simulink model "UPSControl"  (R2025b)
settings: Solver=VariableStepAuto  StartTime=0.0  StopTime=10  FixedStep=Ts  RelTol=1e-3
PostLoadFcn:
  | DataCenterParam;
values from neighbouring files (symbols this model uses):
  generator = struct    [GeneratorParam.m]
  lineInductance = 1e-6    (= 1e-06)    [DataCenterParam.m]    (also in GridParam.m)
  lineResistance = 1e-3    (= 0.001)    [DataCenterParam.m]    (also in GridParam.m)
  loadPower = 5e6    (= 5000000)    [DataCenterParam.m]    (also in LVRT.m; RedundancyAnalysis.m = 10000000)
  machine = struct    [GeneratorParam.m]
  powerTau = 0.005    [DataCenterParam.m]
  Ts = 5e-5    (= 5e-05)    [DataCenterParam.m]    (also in GeneratorParam.m)
  utilizationFactor = 0.45    [DataCenterParam.m]    (also in RedundancyAnalysis.m)
undefined symbols (not defined in the file or in its folder): breaker, ctLimitDelayTime, DiscIntNeverNeededParam, ee_sli_rtmsupport, gcbh, grid, rack, ups
libraries: nesl_utility x96, fl_lib x96, eeGeneralControl x84, ee_lib x80, simulink x68, eeTransforms x30, nesl_utility_internal x16, eeSinusoidalMeasurementV2 x13, slpidlib x12, simulink_extras x12, datacenter_lib x5, batteryecm_lib x4
(part 10 of 13)

== system UPSControl/Server Load/UPS Units/Single UPS/UPS/DC-Link/BESS/DC-DC Converter Controller/Current Reference Generator ==
  VoRef : Inport
  DischargeFlag : Inport  Port=2
  Vo : Inport  Port=3
  I : Inport  Port=4
  Mode : Inport  Port=5
  Add : Sum  Inputs=-+
  Gain : Gain  Gain=droopGain
  Low-Pass Filter (Discrete or Continuous) : eeGeneralControl/Low-Pass Filter (Discrete or Continuous)  K=1  T=0.001  B=inf  A=-inf  init_option=Inherited from block input  x0=0  Ts=-1
  PID Controller : slpidlib/PID Controller  Controller=PI  Form=Parallel  TimeDomain=Discrete-time  UseExternalTs=off  SampleTime=-1  IntegratorMethod=Forward Euler  FilterMethod=Forward Euler  ControllerParametersSource=internal  P=kpDC%500  I=kiDC%500  UseKiTs=off  D=0  UseExternalDerivativeSource=off  N=100  UseFilter=on  TunerSelectOption=Transfer Function Based (PID Tuner App)  InitialConditionSource=internal  InitialConditionForIntegrator=0  InitialConditionForFilter=0  DifferentiatorICPrevScaledInput=0  ExternalReset=rising  TrackingMode=off  Kt=1  LimitOutput=on  SatLimitsSource=internal  UpperSaturationLimit=0  LowerSaturationLimit=-5  LinearizeAsGain=on  AntiWindupMode=clamping  Kb=1  LimitIntegrator=off  UpperIntegratorSaturationLimit=4  LowerIntegratorSaturationLimit=-4  POutMin=[]  POutMax=[]  IOutMin=[]  IOutMax=[]  DOutMin=[]  DOutMax=[]  NOutMin=[]  NOutMax=[]  SumOutMin=[]  SumOutMax=[]  SaturationOutMin=[]  SaturationOutMax=[]  PParamMin=[]  PParamMax=[]  IParamMin=[]  IParamMax=[]  DParamMin=[]  DParamMax=[]  NParamMin=[]  NParamMax=[]  KbParamMin=[]  KbParamMax=[]  KtParamMin=[]  KtParamMax=[]  KbOutMin=[]  KbOutMax=[]  KtOutMin=[]  KtOutMax=[]  IntegratorOutMin=[]  IntegratorOutMax=[]  FilterOutMin=[]  FilterOutMax=[]  SumI1OutMin=[]  SumI1OutMax=[]  SumI2OutMin=[]  SumI2OutMax=[]  SumI3OutMin=[]  SumI3OutMax=[]  SumI4OutMin=[]  SumI4OutMax=[]  SumDOutMin=[]  SumDOutMax=[]  DifferentiatorOutMin=[]  DifferentiatorOutMax=[]  FilterDiffOutCoefMin=[]  FilterDiffOutCoefMax=[]  ReciprocalOutMin=[]  ReciprocalOutMax=[]  SumDenOutMin=[]  SumDenOutMax=[]  SumNumOutMin=[]  SumNumOutMax=[]  DivideOutMin=[]  DivideOutMax=[]  UdiffTsProdOutMin=[]  UdiffTsProdOutMax=[]  NTsProdOutMin=[]  NTsProdOutMax=[]  UintegralTsProdOutMin=[]  UintegralTsProdOutMax=[]  UngainTsProdOutMin=[]  UngainTsProdOutMax=[]  ClampingZeroOutDataTypeStr=Inherit: Inherit via back propagation  ClampingZeroOutMin=[]  ClampingZeroOutMax=[]  FilterDenConstantOutDataTypeStr=Inherit: Inherit via back propagation  FilterDenConstantOutMin=[]  FilterDenConstantOutMax=[]  PCopyOutDataTypeStr=Inherit: Inherit via back propagation  PCopyOutMin=[]  PCopyOutMax=[]  NCopyOutDataTypeStr=Inherit: Inherit via back propagation  NCopyOutMin=[]  NCopyOutMax=[]  IntegratorContinuousStateAttributes=''  IntegratorStateMustResolveToSignalObject=off  IntegratorRTWStateStorageClass=Auto  FilterContinuousStateAttributes=''  FilterStateMustResolveToSignalObject=off  FilterRTWStateStorageClass=Auto  ParallelPVariant=InternalParameters  IdealPVariant=Disabled  IVariant=InternalParameters  DVariant=Disabled  IntegratorVariant=Discrete  SatVariant=Enabled  AWVariant=DiscClampingParallel  PCopyVariant=Disabled  TRVariant=Disabled  FdbkBlocksVariant=Forward  IdealPFdbkVariant=Disabled  SatFdbkVariant=Disabled  DerivativeFilterVariant=Disabled  NVariant=Disabled  NCopyVariant=Disabled_SignalSpec  FilterICVariant=Disabled  IntegratorICVariant=InternalICs  ExternalResetVariant=ExternalReset  TRSumVariant=Passthrough  SumFdbkVariant=Disabled  SumVariant=Sum_PI  TsampFilterVariant=InternalTs  TsampNgainVariant=Passthrough  TsampIntegralVariant=Disabled_SignalSpec  ExternalSaturationOutDataTypeStr=Inherit: Same as second input  DerivativeSourceVariant=Disabled  PreIntVariant=InternalPreInt
  Saturation1 : Saturate  UpperLimit=0  LowerLimit=-10
  Switch1 : Switch  Criteria=u2 > Threshold  SaturateOnIntegerOverflow=off  InputSameDT=off
  Switch3 : Switch  Criteria=u2 > Threshold  SaturateOnIntegerOverflow=off  InputSameDT=off
  i : Outport  VectorParamsAs1DForOutWhenUnconnected=off
  wires:
  Switch1/1 -> Low-Pass Filter (Discrete or Continuous)/1
  Low-Pass Filter (Discrete or Continuous)/1 -> i/1
  Gain/1 -> Saturation1/1
  Switch3/1 -> Switch1/1
  Add/1 -> PID Controller/1, Gain/1
  VoRef/1 -> Add/1
  Vo/1 -> Add/2
  DischargeFlag/1 -> PID Controller/2, Switch1/2
  Mode/1 -> Switch3/2
  Saturation1/1 -> Switch3/1
  PID Controller/1 -> Switch3/3
  I/1 -> Switch1/3

== system UPSControl/Server Load/UPS Units/Single UPS/UPS/DC-Link/BESS/DC-DC Converter Controller/Mode Control ==
  iPFC : Inport
  Vdc : Inport  Port=2
  vBatt : Inport  Port=3
  vPCC : Inport  Port=4
  Breaker : Inport  Port=5
  iCharg : Inport  Port=6
  iBatt : Inport  Port=7
  BMS : Stateflow chart  TreatAsAtomicUnit=on  mask(Microgrid Transition and Dispatch Control){VMaxBatt=vBattMax, VdcRated=baseVoltageDC, iThreshold=vGridMin, iBattTh=10, vThreshold=0.9, VMaxDC=vDCThreshold, VBattNom=vBattMax, initialMode=initialMode}
      mask prompts: VMaxBatt "Maximum Battery Voltage (V)"; VdcRated "Rated DC bus voltage (V)"; iThreshold "Threshold mains current (A)"; iBattTh "Threshold battery current (A)"; vThreshold "Threshold mains voltage (V)"; VMaxDC "Threshold DC Bus Voltage (V)"; VBattNom "Battery nominal voltage (V)"; initialMode "Initial Operating Mode"
      mask help: This subsystem implements the transitions and the corresponding dispatch functions in the microgrid
  Compare To Constant : simulink/Logic and Bit Operations/Compare To Constant  relop===  const=4  OutDataTypeStr=boolean
  Constant : Constant  Value=0.98  OutDataTypeStr=double
  DischargeFlag : Outport
  vOut : Outport  Port=2
  iRef : Outport  Port=3
  droopMode : Outport  Port=4
  Mode : Outport  Port=5
  wires:
  iPFC/1 -> BMS/1(iPFC)
  Vdc/1 -> BMS/2(Vdc)
  vBatt/1 -> BMS/3(VBatt)
  Compare To Constant/1 -> DischargeFlag/1
  Constant/1 -> BMS/4(SOC)
  Breaker/1 -> BMS/5(breakerStatus)
  BMS/1(mode) -> Compare To Constant/1, Mode/1
  vPCC/1 -> BMS/6(VPCC)
  iCharg/1 -> BMS/7(iCharg)
  BMS/3(vOut) -> vOut/1
  BMS/2(iRef) -> iRef/1
  iBatt/1 -> BMS/8(iBatt)
  BMS/4(droopMode) -> droopMode/1

== system UPSControl/Server Load/UPS Units/Single UPS/UPS/Inverter/Filter & Measurements/PLL & Measurements/Measurement1 ==
  u : Inport
  Lead-Lag (Discrete or Continuous) : eeGeneralControl/Lead-Lag (Discrete or Continuous)  T1=0  T2=1e-3  B=inf  A=-inf  init_option=Inherited from block input  x0=0  Ts=Ts
  Vg : Outport
  wires:
  u/1 -> Lead-Lag (Discrete or Continuous)/1
  Lead-Lag (Discrete or Continuous)/1 -> Vg/1

== system UPSControl/Server Load/UPS Units/Single UPS/UPS/Inverter/Filter & Measurements/PLL & Measurements/Measurement2 ==
  u : Inport
  Lead-Lag (Discrete or Continuous) : eeGeneralControl/Lead-Lag (Discrete or Continuous)  T1=0  T2=1e-3  B=inf  A=-inf  init_option=Inherited from block input  x0=0  Ts=Ts
  Vg : Outport
  wires:
  u/1 -> Lead-Lag (Discrete or Continuous)/1
  Lead-Lag (Discrete or Continuous)/1 -> Vg/1

== system UPSControl/Server Load/UPS Units/Single UPS/UPS/Inverter/Filter & Measurements/PLL & Measurements/Subsystem ==
  Vabc : Inport
  Iabc : Inport  Port=2
  Add : Sum  Inputs=+-
  Constant : Constant  Value=pi/2
  Demux : Demux  Outputs=3
  Demux1 : Demux  Outputs=3
  Gain : Gain  Gain=1/frequency
  Gain1 : Gain  Gain=1/sqrt(2)
  Park Transform : eeTransforms/Park Transform  AxisAlignment=Q-axis  PowerInvariant=off
  Park Transform1 : eeTransforms/Park Transform  AxisAlignment=D-axis  PowerInvariant=off
  Scope : Scope  NumInputPorts=2
      settings: ActiveDisplayYMinimum=-0.205092135439717  ActiveDisplayYMaximum=1.5105061212865092  DataLoggingVariableName=ScopeData5
  Scope1 : Scope  NumInputPorts=2
      settings: ActiveDisplayYMinimum=-0.28974456970762869  ActiveDisplayYMaximum=0.89280252648921143  DataLoggingVariableName=ScopeData10
  Scope2 : Scope  NumInputPorts=2
      settings: ActiveDisplayYMinimum=-1  ActiveDisplayYMaximum=1  DataLoggingVariableName=ScopeData33
  Scope3 : Scope
      settings: ActiveDisplayYMinimum=-0.19602223868392757  ActiveDisplayYMaximum=1.7642001481553486  DataLoggingVariableName=ScopeData34
  "Sinusoidal Measurement (PLL, Three-Phase)" : eeSinusoidalMeasurementV2/Sinusoidal Measurement (PLL, Three-Phase)  InputFilter=on  InputNormalization=off  Kp_LF=40  Ki_LF=1000  F0=frequency  Theta0=0  Ts=Ts
  Terminator : Terminator
  Terminator1 : Terminator
  mag : Outport
  freq : Outport  Port=2
  angle : Outport  Port=3
  Vd : Outport  Port=4
  Vq : Outport  Port=5
  Id1 : Outport  Port=6
  Iq1 : Outport  Port=7
  wires:
  Iabc/1 -> Park Transform1/1
  Demux1/3 -> Terminator1/1
  Demux1/2 -> Scope1/2, Iq1/1
  Demux1/1 -> Scope1/1, Id1/1
  Park Transform1/1 -> Demux1/1
  "Sinusoidal Measurement (PLL, Three-Phase)"/3 -> Gain1/1
  "Sinusoidal Measurement (PLL, Three-Phase)"/1 -> Gain/1
  "Sinusoidal Measurement (PLL, Three-Phase)"/2 -> Park Transform/2, angle/1, Add/1
  Demux/2 -> Vq/1, Scope/2
  Demux/1 -> Vd/1, Scope/1
  Park Transform/1 -> Demux/1
  Vabc/1 -> Park Transform/1, "Sinusoidal Measurement (PLL, Three-Phase)"/1
  Demux/3 -> Terminator/1
  Gain/1 -> Scope2/1, freq/1
  Gain1/1 -> Scope3/1, mag/1
  Constant/1 -> Add/2
  Add/1 -> Park Transform1/2

== system UPSControl/Server Load/UPS Units/Single UPS/UPS/Inverter/Inverter Controller/Current Limiter/Current Limiter ==
  Igd : Inport
  Igq : Inport  Port=2
  Current Saturation : Subsystem  VariantControl=Current Saturation
  Virtual Impedance : Subsystem  VariantControl=Virtual Impedance
  delVd : Outport
  delVq : Outport  Port=2
  Idmax : Outport  Port=3
  Iqmax : Outport  Port=4

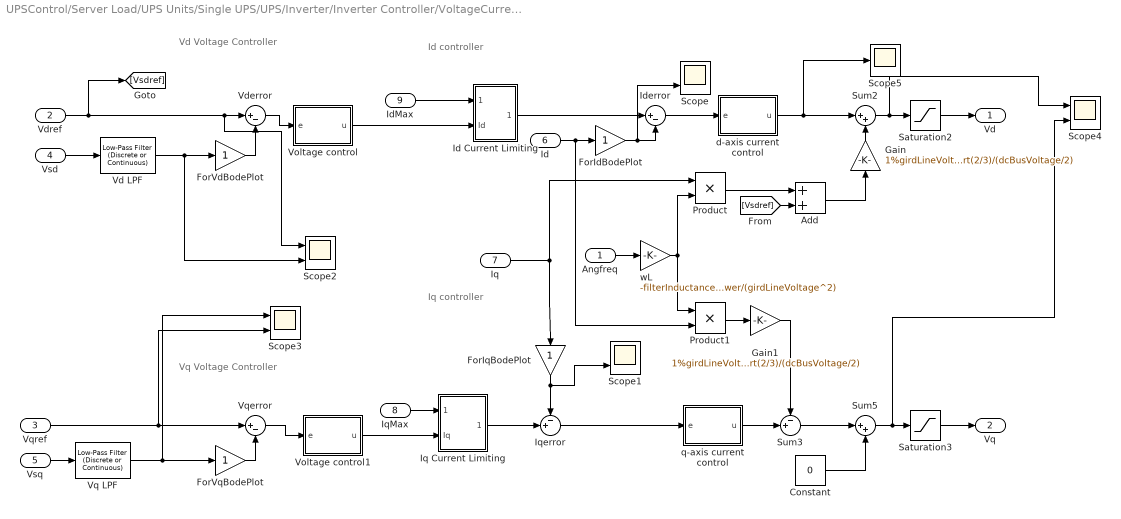
== system UPSControl/Server Load/UPS Units/Single UPS/UPS/Inverter/Inverter Controller/VoltageCurrentControl/Controller ==
  note: Vq Voltage Controller
  note: Iq controller
  note: Vd Voltage Controller
  note: Id controller
  Angfreq : Inport
  Vdref : Inport  Port=2
  Vqref : Inport  Port=3
  Vsd : Inport  Port=4
  Vsq : Inport  Port=5
  Id : Inport  Port=6
  Iq : Inport  Port=7
  IqMax : Inport  Port=8
  IdMax : Inport  Port=9
  Add : Sum
  Constant : Constant  Value=0  SampleTime=currentControlTs
  ForIdBodePlot : Gain
  ForIqBodePlot : Gain
  ForVdBodePlot : Gain
  ForVqBodePlot : Gain
  Gain : Gain  Gain=1%girdLineVoltage*sqrt(2/3)/(dcBusVoltage/2)
  Gain1 : Gain  Gain=1%girdLineVoltage*sqrt(2/3)/(dcBusVoltage/2)
  Id Current Limiting : Subsystem
  Iderror : Sum  Inputs=|+-
  Iq Current Limiting : Subsystem
  Iqerror : Sum  Inputs=-+|
  Product : Product
  Product1 : Product
  Saturation2 : Saturate  UpperLimit=1.5  LowerLimit=-1.5
  Saturation3 : Saturate  UpperLimit=1.5  LowerLimit=-1.5
  Scope{,1..4} (5 alike) : Scope  NumInputPorts=2
      Scope settings: ActiveDisplayYMinimum=-1.8047219913264509  ActiveDisplayYMaximum=2.2005246657029387
      Scope1 settings: ActiveDisplayYMinimum=-0.5206159009733754  ActiveDisplayYMaximum=0.33911481242712255
      Scope2 settings: ActiveDisplayYMinimum=0.98739217845302751  ActiveDisplayYMaximum=1.0346201805103583
      Scope3 settings: ActiveDisplayYMinimum=-1.1546814525903495  ActiveDisplayYMaximum=0.39213307331314629
      Scope4 settings: ActiveDisplayYMinimum=-0.18956095761758107  ActiveDisplayYMaximum=1.4204991580589943  DataLoggingVariableName=ScopeData41
  Scope5 : Scope
      settings: ActiveDisplayYMinimum=-1  ActiveDisplayYMaximum=1  DataLoggingVariableName=ScopeData42
  Sum2 : Sum  Inputs=|++
  Sum3 : Sum  Inputs=-+|
  Sum5 : Sum  Inputs=|++
  Vd LPF : eeGeneralControl/Low-Pass Filter (Discrete or Continuous)  K=1  T=vdvqLPFTimeConst  B=inf  A=-inf  init_option=Specify as parameter  x0=0  Ts=voltControlTs
  Vderror : Sum  Inputs=|+-
  Voltage control : Subsystem
  Voltage control1 : Subsystem
  Vq LPF : eeGeneralControl/Low-Pass Filter (Discrete or Continuous)  K=1  T=vdvqLPFTimeConst  B=inf  A=-inf  init_option=Inherited from block input  x0=0  Ts=voltControlTs
  Vqerror : Sum  Inputs=|+-
  d-axis current control : Subsystem
  q-axis current control : Subsystem
  wL : Gain  Gain=-filterInductance*power/(girdLineVoltage^2)
  Vd : Outport  VectorParamsAs1DForOutWhenUnconnected=off
  Vq : Outport  Port=2  VectorParamsAs1DForOutWhenUnconnected=off
  wires:
  Vdref/1 -> [Vsdref], Vderror/1, Scope2/1
  Vq LPF/1 -> ForVqBodePlot/1, Scope3/1
  Vd LPF/1 -> ForVdBodePlot/1, Scope2/2
  ForIqBodePlot/1 -> Iqerror/1, Scope1/2
  ForIdBodePlot/1 -> Iderror/2, Scope/2
  ForVqBodePlot/1 -> Vqerror/2
  ForVdBodePlot/1 -> Vderror/2
  Vsd/1 -> Vd LPF/1
  Gain/1 -> Sum2/2
  Add/1 -> Gain/1
  [Vsdref] -> Add/2
  Gain1/1 -> Sum3/1
  Vqerror/1 -> Voltage control1/1(e)
  Vqref/1 -> Vqerror/1, Scope3/2
  Vderror/1 -> Voltage control/1(e)
  Id/1 -> ForIdBodePlot/1, Product1/2
  Vsq/1 -> Vq LPF/1
  Sum5/1 -> Scope4/2, Saturation3/1
  Sum3/1 -> Sum5/1
  q-axis current control/1(u) -> Sum3/2
  Sum2/1 -> Scope4/1, Saturation2/1
  d-axis current control/1(u) -> Scope5/1, Sum2/1
  Product/1 -> Add/1
  Product1/1 -> Gain1/1
  Saturation2/1 -> Vd/1
  Saturation3/1 -> Vq/1
  Iderror/1 -> d-axis current control/1(e)
  Constant/1 -> Sum5/2
  Angfreq/1 -> wL/1
  wL/1 -> Product/2, Product1/1
  Iqerror/1 -> q-axis current control/1(e)
  Iq/1 -> Product/1, ForIqBodePlot/1
  IdMax/1 -> Id Current Limiting/1(Imax)
  IqMax/1 -> Iq Current Limiting/1(Imax)
  Voltage control/1(u) -> Id Current Limiting/2(Id)
  Id Current Limiting/1(Idref) -> Iderror/1
  Voltage control1/1(u) -> Iq Current Limiting/2(Iq)
  Iq Current Limiting/1(Iqref) -> Iqerror/2

== system UPSControl/Server Load/UPS Units/Single UPS/UPS/Inverter/Inverter Controller/VoltageCurrentControl/Modulation Signal ==
  Vd : Inport
  Vq : Inport  Port=2
  Angle : Inport  Port=3
  Constant : Constant  Value=0
  Constant1 : Constant  Value=1.05
  Inverse Park Transform : eeTransforms/Inverse Park Transform  AxisAlignment=D-axis  PowerInvariant=off
  Mux1 : Mux  Inputs=3
  Saturation : Saturate  UpperLimit=1.2  LowerLimit=-1.2
  Saturation1 : Saturate
  Saturation2 : Saturate  UpperLimit=1  LowerLimit=-1
  Scope : Scope  NumInputPorts=2
      settings: ActiveDisplayYMinimum=-1  ActiveDisplayYMaximum=1  DataLoggingVariableName=ScopeData9
  Scope1 : Scope
      settings: ActiveDisplayYMinimum=-1  ActiveDisplayYMaximum=1
  Scope2 : Scope
      settings: ActiveDisplayYMinimum=-1.25  ActiveDisplayYMaximum=1.25  DataLoggingVariableName=ScopeData47
  mabc : Outport  VectorParamsAs1DForOutWhenUnconnected=off
  wires:
  Vq/1 -> Saturation1/1, Scope/2
  Vd/1 -> Saturation/1, Scope/1
  Constant/1 -> Mux1/3
  Saturation2/1 -> Scope2/1, mabc/1
  Angle/1 -> Inverse Park Transform/2, Scope1/1
  Mux1/1 -> Inverse Park Transform/1
  Inverse Park Transform/1 -> Saturation2/1
  Saturation/1 -> Mux1/1
  Saturation1/1 -> Mux1/2

== system UPSControl/Server Load/UPS Units/Single UPS/UPS/Rectifier/PFC Rectifier Controller/Current Controller/Id and Iq Controller ==
  idRef : Inport
  iqRef : Inport  Port=2
  IdSens : Inport  Port=3
  iqSens : Inport  Port=4
  vd : Inport  Port=5
  vq : Inport  Port=6
  Reset : Inport  Port=7
  Constant4 : Constant  Value=0  SampleTime=Ts
  Gain1 : Gain  Gain=2*1*pi*Freq*L/BaseImpedance
  Gain2 : Gain  Gain=2*1*pi*Freq*L/BaseImpedance
  IdPID : slpidlib/PID Controller  Controller=PID  Form=Parallel  TimeDomain=Discrete-time  UseExternalTs=off  SampleTime=Ts  IntegratorMethod=Forward Euler  FilterMethod=Forward Euler  ControllerParametersSource=internal  P=KpdCurrent  I=KidCurrent  UseKiTs=off  D=KddCurrent  UseExternalDerivativeSource=off  N=NdCurrent  UseFilter=on  TunerSelectOption=Transfer Function Based (PID Tuner App)  InitialConditionSource=internal  InitialConditionForIntegrator=0  InitialConditionForFilter=0  DifferentiatorICPrevScaledInput=0  ExternalReset=falling  TrackingMode=off  Kt=1  LimitOutput=on  SatLimitsSource=internal  UpperSaturationLimit=IdControlUpperLimit  LowerSaturationLimit=IdControlLowerLimit  LinearizeAsGain=on  AntiWindupMode=clamping  Kb=1  LimitIntegrator=on  UpperIntegratorSaturationLimit=IdControlUpperLimit  LowerIntegratorSaturationLimit=IdControlLowerLimit  POutMin=[]  POutMax=[]  IOutMin=[]  IOutMax=[]  DOutMin=[]  DOutMax=[]  NOutMin=[]  NOutMax=[]  SumOutMin=[]  SumOutMax=[]  SaturationOutMin=[]  SaturationOutMax=[]  PParamMin=[]  PParamMax=[]  IParamMin=[]  IParamMax=[]  DParamMin=[]  DParamMax=[]  NParamMin=[]  NParamMax=[]  KbParamMin=[]  KbParamMax=[]  KtParamMin=[]  KtParamMax=[]  KbOutMin=[]  KbOutMax=[]  KtOutMin=[]  KtOutMax=[]  IntegratorOutMin=[]  IntegratorOutMax=[]  FilterOutMin=[]  FilterOutMax=[]  SumI1OutMin=[]  SumI1OutMax=[]  SumI2OutMin=[]  SumI2OutMax=[]  SumI3OutMin=[]  SumI3OutMax=[]  SumI4OutMin=[]  SumI4OutMax=[]  SumDOutMin=[]  SumDOutMax=[]  DifferentiatorOutMin=[]  DifferentiatorOutMax=[]  FilterDiffOutCoefMin=[]  FilterDiffOutCoefMax=[]  ReciprocalOutMin=[]  ReciprocalOutMax=[]  SumDenOutMin=[]  SumDenOutMax=[]  SumNumOutMin=[]  SumNumOutMax=[]  DivideOutMin=[]  DivideOutMax=[]  UdiffTsProdOutMin=[]  UdiffTsProdOutMax=[]  NTsProdOutMin=[]  NTsProdOutMax=[]  UintegralTsProdOutMin=[]  UintegralTsProdOutMax=[]  UngainTsProdOutMin=[]  UngainTsProdOutMax=[]  ClampingZeroOutDataTypeStr=Inherit: Inherit via back propagation  ClampingZeroOutMin=[]  ClampingZeroOutMax=[]  FilterDenConstantOutDataTypeStr=Inherit: Inherit via back propagation  FilterDenConstantOutMin=[]  FilterDenConstantOutMax=[]  PCopyOutDataTypeStr=Inherit: Inherit via back propagation  PCopyOutMin=[]  PCopyOutMax=[]  NCopyOutDataTypeStr=Inherit: Inherit via back propagation  NCopyOutMin=[]  NCopyOutMax=[]  IntegratorContinuousStateAttributes=''  IntegratorStateMustResolveToSignalObject=off  IntegratorRTWStateStorageClass=Auto  FilterContinuousStateAttributes=''  FilterStateMustResolveToSignalObject=off  FilterRTWStateStorageClass=Auto  ParallelPVariant=InternalParameters  IdealPVariant=Disabled  IVariant=InternalParameters  DVariant=InternalParameters  IntegratorVariant=Discrete  SatVariant=Enabled  AWVariant=DiscClampingParallel  PCopyVariant=Disabled  TRVariant=Disabled  FdbkBlocksVariant=Forward  IdealPFdbkVariant=Disabled  SatFdbkVariant=Disabled  DerivativeFilterVariant=ForwardEulerFilter  NVariant=InternalParameters  NCopyVariant=Disabled  FilterICVariant=InternalICsFilter  IntegratorICVariant=InternalICs  ExternalResetVariant=ExternalReset  TRSumVariant=Passthrough  SumFdbkVariant=Disabled  SumVariant=Sum_PID  TsampFilterVariant=InternalTs  TsampNgainVariant=Passthrough  TsampIntegralVariant=Disabled_SignalSpec  ExternalSaturationOutDataTypeStr=Inherit: Same as second input  DerivativeSourceVariant=ErrorSignal  PreIntVariant=InternalPreInt
  IqPID : slpidlib/PID Controller  Controller=PID  Form=Parallel  TimeDomain=Discrete-time  UseExternalTs=off  SampleTime=Ts  IntegratorMethod=Forward Euler  FilterMethod=Forward Euler  ControllerParametersSource=internal  P=KpqCurrent  I=KiqCurrent  UseKiTs=off  D=KdqCurrent  UseExternalDerivativeSource=off  N=NdCurrent  UseFilter=on  TunerSelectOption=Transfer Function Based (PID Tuner App)  InitialConditionSource=internal  InitialConditionForIntegrator=0  InitialConditionForFilter=0  DifferentiatorICPrevScaledInput=0  ExternalReset=falling  TrackingMode=off  Kt=1  LimitOutput=on  SatLimitsSource=internal  UpperSaturationLimit=IqControlUpperLimit  LowerSaturationLimit=IqControlLowerLimit  LinearizeAsGain=on  AntiWindupMode=clamping  Kb=1  LimitIntegrator=on  UpperIntegratorSaturationLimit=IqControlUpperLimit  LowerIntegratorSaturationLimit=IqControlLowerLimit  POutMin=[]  POutMax=[]  IOutMin=[]  IOutMax=[]  DOutMin=[]  DOutMax=[]  NOutMin=[]  NOutMax=[]  SumOutMin=[]  SumOutMax=[]  SaturationOutMin=[]  SaturationOutMax=[]  PParamMin=[]  PParamMax=[]  IParamMin=[]  IParamMax=[]  DParamMin=[]  DParamMax=[]  NParamMin=[]  NParamMax=[]  KbParamMin=[]  KbParamMax=[]  KtParamMin=[]  KtParamMax=[]  KbOutMin=[]  KbOutMax=[]  KtOutMin=[]  KtOutMax=[]  IntegratorOutMin=[]  IntegratorOutMax=[]  FilterOutMin=[]  FilterOutMax=[]  SumI1OutMin=[]  SumI1OutMax=[]  SumI2OutMin=[]  SumI2OutMax=[]  SumI3OutMin=[]  SumI3OutMax=[]  SumI4OutMin=[]  SumI4OutMax=[]  SumDOutMin=[]  SumDOutMax=[]  DifferentiatorOutMin=[]  DifferentiatorOutMax=[]  FilterDiffOutCoefMin=[]  FilterDiffOutCoefMax=[]  ReciprocalOutMin=[]  ReciprocalOutMax=[]  SumDenOutMin=[]  SumDenOutMax=[]  SumNumOutMin=[]  SumNumOutMax=[]  DivideOutMin=[]  DivideOutMax=[]  UdiffTsProdOutMin=[]  UdiffTsProdOutMax=[]  NTsProdOutMin=[]  NTsProdOutMax=[]  UintegralTsProdOutMin=[]  UintegralTsProdOutMax=[]  UngainTsProdOutMin=[]  UngainTsProdOutMax=[]  ClampingZeroOutDataTypeStr=Inherit: Inherit via back propagation  ClampingZeroOutMin=[]  ClampingZeroOutMax=[]  FilterDenConstantOutDataTypeStr=Inherit: Inherit via back propagation  FilterDenConstantOutMin=[]  FilterDenConstantOutMax=[]  PCopyOutDataTypeStr=Inherit: Inherit via back propagation  PCopyOutMin=[]  PCopyOutMax=[]  NCopyOutDataTypeStr=Inherit: Inherit via back propagation  NCopyOutMin=[]  NCopyOutMax=[]  IntegratorContinuousStateAttributes=''  IntegratorStateMustResolveToSignalObject=off  IntegratorRTWStateStorageClass=Auto  FilterContinuousStateAttributes=''  FilterStateMustResolveToSignalObject=off  FilterRTWStateStorageClass=Auto  ParallelPVariant=InternalParameters  IdealPVariant=Disabled  IVariant=InternalParameters  DVariant=InternalParameters  IntegratorVariant=Discrete  SatVariant=Enabled  AWVariant=DiscClampingParallel  PCopyVariant=Disabled  TRVariant=Disabled  FdbkBlocksVariant=Forward  IdealPFdbkVariant=Disabled  SatFdbkVariant=Disabled  DerivativeFilterVariant=ForwardEulerFilter  NVariant=InternalParameters  NCopyVariant=Disabled  FilterICVariant=InternalICsFilter  IntegratorICVariant=InternalICs  ExternalResetVariant=ExternalReset  TRSumVariant=Passthrough  SumFdbkVariant=Disabled  SumVariant=Sum_PID  TsampFilterVariant=InternalTs  TsampNgainVariant=Passthrough  TsampIntegralVariant=Disabled_SignalSpec  ExternalSaturationOutDataTypeStr=Inherit: Same as second input  DerivativeSourceVariant=ErrorSignal  PreIntVariant=InternalPreInt
  Mux1 : Mux  Inputs=3
  Sum1 : Sum  Inputs=|+-
  Sum2 : Sum  Inputs=|+-+
  Sum4 : Sum  Inputs=|--+
  Sum5 : Sum  Inputs=|+-
  vdqoRef : Outport
  IdCntrlError : Outport  Port=2
  IqCntrlError : Outport  Port=3
  wires:
  iqRef/1 -> Sum5/1
  Mux1/1 -> vdqoRef/1
  idRef/1 -> Sum1/1
  IqPID/1 -> Sum4/2
  IdSens/1 -> Gain1/1, Sum1/2
  Sum1/1 -> IdPID/1, IdCntrlError/1
  vd/1 -> Sum2/1
  IdPID/1 -> Sum2/2
  Gain2/1 -> Sum2/3
  Gain1/1 -> Sum4/1
  vq/1 -> Sum4/3
  iqSens/1 -> Gain2/1, Sum5/2
  Sum2/1 -> Mux1/1
  Sum4/1 -> Mux1/2
  Sum5/1 -> IqPID/1, IqCntrlError/1
  Constant4/1 -> Mux1/3
  Reset/1 -> IqPID/2, IdPID/2

== system UPSControl/Server Load/UPS Units/Single UPS/UPS/Rectifier/PFC Rectifier Controller/DC Voltage Controller and Current Reference/Iq Reference ==
  V_mag : Inport
  Q_ref : Inport  Port=2
  Divide2 : Product  Inputs=*/
  iq_ref : Outport
  wires:
  V_mag/1 -> Divide2/2
  Q_ref/1 -> Divide2/1
  Divide2/1 -> iq_ref/1

== system UPSControl/Server Load/UPS Units/Single UPS/UPS/Rectifier/PFC Rectifier Controller/DC Voltage Controller and Current Reference/Voltage Controller ==
  Vdcref : Inport
  Vdcmeas : Inport  Port=2
  Reset : Inport  Port=3
  Gain : Gain  Gain=1/BaseVdc
  Saturation : Saturate  UpperLimit=IdRefUpperLimit  LowerLimit=0
  Sum : Sum  Inputs=|+-
  Voltage control : Subsystem
  Id : Outport
  wires:
  Sum/1 -> Gain/1
  Gain/1 -> Voltage control/1(e)
  Vdcmeas/1 -> Sum/2
  Vdcref/1 -> Sum/1
  Voltage control/1(u) -> Saturation/1
  Saturation/1 -> Id/1
  Reset/1 -> Voltage control/2(Reset)

== system UPSControl/Server Load/UPS Units/Three UPS Parallel/UPS1/DC-Link/BESS/DC-DC Converter Controller/Current Reference Generator ==
  VoRef : Inport
  DischargeFlag : Inport  Port=2
  Vo : Inport  Port=3
  I : Inport  Port=4
  Mode : Inport  Port=5
  Add : Sum  Inputs=-+
  Gain : Gain  Gain=droopGain
  Low-Pass Filter (Discrete or Continuous) : eeGeneralControl/Low-Pass Filter (Discrete or Continuous)  K=1  T=0.001  B=inf  A=-inf  init_option=Inherited from block input  x0=0  Ts=-1
  PID Controller : slpidlib/PID Controller  Controller=PI  Form=Parallel  TimeDomain=Discrete-time  UseExternalTs=off  SampleTime=-1  IntegratorMethod=Forward Euler  FilterMethod=Forward Euler  ControllerParametersSource=internal  P=kpDC  I=kiDC*10  UseKiTs=off  D=0  UseExternalDerivativeSource=off  N=100  UseFilter=on  TunerSelectOption=Transfer Function Based (PID Tuner App)  InitialConditionSource=internal  InitialConditionForIntegrator=0  InitialConditionForFilter=0  DifferentiatorICPrevScaledInput=0  ExternalReset=rising  TrackingMode=off  Kt=1  LimitOutput=on  SatLimitsSource=internal  UpperSaturationLimit=0  LowerSaturationLimit=-5  LinearizeAsGain=on  AntiWindupMode=clamping  Kb=1  LimitIntegrator=off  UpperIntegratorSaturationLimit=4  LowerIntegratorSaturationLimit=-4  POutMin=[]  POutMax=[]  IOutMin=[]  IOutMax=[]  DOutMin=[]  DOutMax=[]  NOutMin=[]  NOutMax=[]  SumOutMin=[]  SumOutMax=[]  SaturationOutMin=[]  SaturationOutMax=[]  PParamMin=[]  PParamMax=[]  IParamMin=[]  IParamMax=[]  DParamMin=[]  DParamMax=[]  NParamMin=[]  NParamMax=[]  KbParamMin=[]  KbParamMax=[]  KtParamMin=[]  KtParamMax=[]  KbOutMin=[]  KbOutMax=[]  KtOutMin=[]  KtOutMax=[]  IntegratorOutMin=[]  IntegratorOutMax=[]  FilterOutMin=[]  FilterOutMax=[]  SumI1OutMin=[]  SumI1OutMax=[]  SumI2OutMin=[]  SumI2OutMax=[]  SumI3OutMin=[]  SumI3OutMax=[]  SumI4OutMin=[]  SumI4OutMax=[]  SumDOutMin=[]  SumDOutMax=[]  DifferentiatorOutMin=[]  DifferentiatorOutMax=[]  FilterDiffOutCoefMin=[]  FilterDiffOutCoefMax=[]  ReciprocalOutMin=[]  ReciprocalOutMax=[]  SumDenOutMin=[]  SumDenOutMax=[]  SumNumOutMin=[]  SumNumOutMax=[]  DivideOutMin=[]  DivideOutMax=[]  UdiffTsProdOutMin=[]  UdiffTsProdOutMax=[]  NTsProdOutMin=[]  NTsProdOutMax=[]  UintegralTsProdOutMin=[]  UintegralTsProdOutMax=[]  UngainTsProdOutMin=[]  UngainTsProdOutMax=[]  ClampingZeroOutDataTypeStr=Inherit: Inherit via back propagation  ClampingZeroOutMin=[]  ClampingZeroOutMax=[]  FilterDenConstantOutDataTypeStr=Inherit: Inherit via back propagation  FilterDenConstantOutMin=[]  FilterDenConstantOutMax=[]  PCopyOutDataTypeStr=Inherit: Inherit via back propagation  PCopyOutMin=[]  PCopyOutMax=[]  NCopyOutDataTypeStr=Inherit: Inherit via back propagation  NCopyOutMin=[]  NCopyOutMax=[]  IntegratorContinuousStateAttributes=''  IntegratorStateMustResolveToSignalObject=off  IntegratorRTWStateStorageClass=Auto  FilterContinuousStateAttributes=''  FilterStateMustResolveToSignalObject=off  FilterRTWStateStorageClass=Auto  ParallelPVariant=InternalParameters  IdealPVariant=Disabled  IVariant=InternalParameters  DVariant=Disabled  IntegratorVariant=Discrete  SatVariant=Enabled  AWVariant=DiscClampingParallel  PCopyVariant=Disabled  TRVariant=Disabled  FdbkBlocksVariant=Forward  IdealPFdbkVariant=Disabled  SatFdbkVariant=Disabled  DerivativeFilterVariant=Disabled  NVariant=Disabled  NCopyVariant=Disabled_SignalSpec  FilterICVariant=Disabled  IntegratorICVariant=InternalICs  ExternalResetVariant=ExternalReset  TRSumVariant=Passthrough  SumFdbkVariant=Disabled  SumVariant=Sum_PI  TsampFilterVariant=InternalTs  TsampNgainVariant=Passthrough  TsampIntegralVariant=Disabled_SignalSpec  ExternalSaturationOutDataTypeStr=Inherit: Same as second input  DerivativeSourceVariant=Disabled  PreIntVariant=InternalPreInt
  Saturation1 : Saturate  UpperLimit=0  LowerLimit=-10
  Switch1 : Switch  Criteria=u2 > Threshold  SaturateOnIntegerOverflow=off  InputSameDT=off
  Switch3 : Switch  Criteria=u2 > Threshold  SaturateOnIntegerOverflow=off  InputSameDT=off
  i : Outport  VectorParamsAs1DForOutWhenUnconnected=off
  wires:
  Switch1/1 -> Low-Pass Filter (Discrete or Continuous)/1
  Low-Pass Filter (Discrete or Continuous)/1 -> i/1
  Gain/1 -> Saturation1/1
  Switch3/1 -> Switch1/1
  Add/1 -> PID Controller/1, Gain/1
  VoRef/1 -> Add/1
  Vo/1 -> Add/2
  DischargeFlag/1 -> PID Controller/2, Switch1/2
  Mode/1 -> Switch3/2
  Saturation1/1 -> Switch3/1
  PID Controller/1 -> Switch3/3
  I/1 -> Switch1/3

== system UPSControl/Server Load/UPS Units/Three UPS Parallel/UPS1/DC-Link/BESS/DC-DC Converter Controller/Mode Control ==
  iPFC : Inport
  Vdc : Inport  Port=2
  vBatt : Inport  Port=3
  vPCC : Inport  Port=4
  Breaker : Inport  Port=5
  iCharg : Inport  Port=6
  iBatt : Inport  Port=7
  BMS : Stateflow chart  TreatAsAtomicUnit=on  mask(Microgrid Transition and Dispatch Control){VMaxBatt=vBattMax, VdcRated=baseVoltageDC, iThreshold=vGridMin, iBattTh=10, vThreshold=0.9, VMaxDC=vDCThreshold, VBattNom=vBattMax, initialMode=initialMode}
      mask prompts: VMaxBatt "Maximum Battery Voltage (V)"; VdcRated "Rated DC bus voltage (V)"; iThreshold "Threshold mains current (A)"; iBattTh "Threshold battery current (A)"; vThreshold "Threshold mains voltage (V)"; VMaxDC "Threshold DC Bus Voltage (V)"; VBattNom "Battery nominal voltage (V)"; initialMode "Initial Operating Mode"
      mask help: This subsystem implements the transitions and the corresponding dispatch functions in the microgrid
  Compare To Constant : simulink/Logic and Bit Operations/Compare To Constant  relop===  const=4  OutDataTypeStr=boolean
  Constant : Constant  Value=0.98  OutDataTypeStr=double
  DischargeFlag : Outport
  vOut : Outport  Port=2
  iRef : Outport  Port=3
  droopMode : Outport  Port=4
  Mode : Outport  Port=5
  wires:
  iPFC/1 -> BMS/1(iPFC)
  Vdc/1 -> BMS/2(Vdc)
  vBatt/1 -> BMS/3(VBatt)
  Compare To Constant/1 -> DischargeFlag/1
  Constant/1 -> BMS/4(SOC)
  Breaker/1 -> BMS/5(breakerStatus)
  BMS/1(mode) -> Compare To Constant/1, Mode/1
  vPCC/1 -> BMS/6(VPCC)
  iCharg/1 -> BMS/7(iCharg)
  BMS/3(vOut) -> vOut/1
  BMS/2(iRef) -> iRef/1
  iBatt/1 -> BMS/8(iBatt)
  BMS/4(droopMode) -> droopMode/1

== system UPSControl/Server Load/UPS Units/Three UPS Parallel/UPS1/Inverter/Filter & Measurements/PLL & Measurements/Measurement1 ==
  u : Inport
  Lead-Lag (Discrete or Continuous) : eeGeneralControl/Lead-Lag (Discrete or Continuous)  T1=0  T2=1e-3  B=inf  A=-inf  init_option=Inherited from block input  x0=0  Ts=Ts
  Vg : Outport
  wires:
  u/1 -> Lead-Lag (Discrete or Continuous)/1
  Lead-Lag (Discrete or Continuous)/1 -> Vg/1

== system UPSControl/Server Load/UPS Units/Three UPS Parallel/UPS1/Inverter/Filter & Measurements/PLL & Measurements/Measurement2 ==
  u : Inport
  Lead-Lag (Discrete or Continuous) : eeGeneralControl/Lead-Lag (Discrete or Continuous)  T1=0  T2=1e-3  B=inf  A=-inf  init_option=Inherited from block input  x0=0  Ts=Ts
  Vg : Outport
  wires:
  u/1 -> Lead-Lag (Discrete or Continuous)/1
  Lead-Lag (Discrete or Continuous)/1 -> Vg/1

== system UPSControl/Server Load/UPS Units/Three UPS Parallel/UPS1/Inverter/Filter & Measurements/PLL & Measurements/Subsystem ==
  Vabc : Inport
  Iabc : Inport  Port=2
  Add : Sum  Inputs=+-
  Constant : Constant  Value=pi/2
  Demux : Demux  Outputs=3
  Demux1 : Demux  Outputs=3
  Gain : Gain  Gain=1/frequency
  Gain1 : Gain  Gain=1/sqrt(2)
  Park Transform : eeTransforms/Park Transform  AxisAlignment=Q-axis  PowerInvariant=off
  Park Transform1 : eeTransforms/Park Transform  AxisAlignment=D-axis  PowerInvariant=off
  Scope : Scope  NumInputPorts=2
      settings: ActiveDisplayYMinimum=-0.205092135439717  ActiveDisplayYMaximum=1.5105061212865092  DataLoggingVariableName=ScopeData5
  Scope1 : Scope  NumInputPorts=2
      settings: ActiveDisplayYMinimum=-0.28974456970762869  ActiveDisplayYMaximum=0.89280252648921143  DataLoggingVariableName=ScopeData10
  Scope2 : Scope  NumInputPorts=2
      settings: ActiveDisplayYMinimum=-1  ActiveDisplayYMaximum=1  DataLoggingVariableName=ScopeData33
  Scope3 : Scope
      settings: ActiveDisplayYMinimum=-0.19602223868392757  ActiveDisplayYMaximum=1.7642001481553486  DataLoggingVariableName=ScopeData34
  "Sinusoidal Measurement (PLL, Three-Phase)" : eeSinusoidalMeasurementV2/Sinusoidal Measurement (PLL, Three-Phase)  InputFilter=on  InputNormalization=off  Kp_LF=40  Ki_LF=1000  F0=frequency  Theta0=0  Ts=Ts
  Terminator : Terminator
  Terminator1 : Terminator
  mag : Outport
  freq : Outport  Port=2
  angle : Outport  Port=3
  Vd : Outport  Port=4
  Vq : Outport  Port=5
  Id1 : Outport  Port=6
  Iq1 : Outport  Port=7
  wires:
  Iabc/1 -> Park Transform1/1
  Demux1/3 -> Terminator1/1
  Demux1/2 -> Scope1/2, Iq1/1
  Demux1/1 -> Scope1/1, Id1/1
  Park Transform1/1 -> Demux1/1
  "Sinusoidal Measurement (PLL, Three-Phase)"/3 -> Gain1/1
  "Sinusoidal Measurement (PLL, Three-Phase)"/1 -> Gain/1
  "Sinusoidal Measurement (PLL, Three-Phase)"/2 -> Park Transform/2, angle/1, Add/1
  Demux/2 -> Vq/1, Scope/2
  Demux/1 -> Vd/1, Scope/1
  Park Transform/1 -> Demux/1
  Vabc/1 -> Park Transform/1, "Sinusoidal Measurement (PLL, Three-Phase)"/1
  Demux/3 -> Terminator/1
  Gain/1 -> Scope2/1, freq/1
  Gain1/1 -> Scope3/1, mag/1
  Constant/1 -> Add/2
  Add/1 -> Park Transform1/2

== system UPSControl/Server Load/UPS Units/Three UPS Parallel/UPS1/Inverter/Inverter Controller/Current Limiter/Current Limiter ==
  Igd : Inport
  Igq : Inport  Port=2
  Current Saturation : Subsystem  VariantControl=Current Saturation
  Virtual Impedance : Subsystem  VariantControl=Virtual Impedance
  delVd : Outport
  delVq : Outport  Port=2
  Idmax : Outport  Port=3
  Iqmax : Outport  Port=4

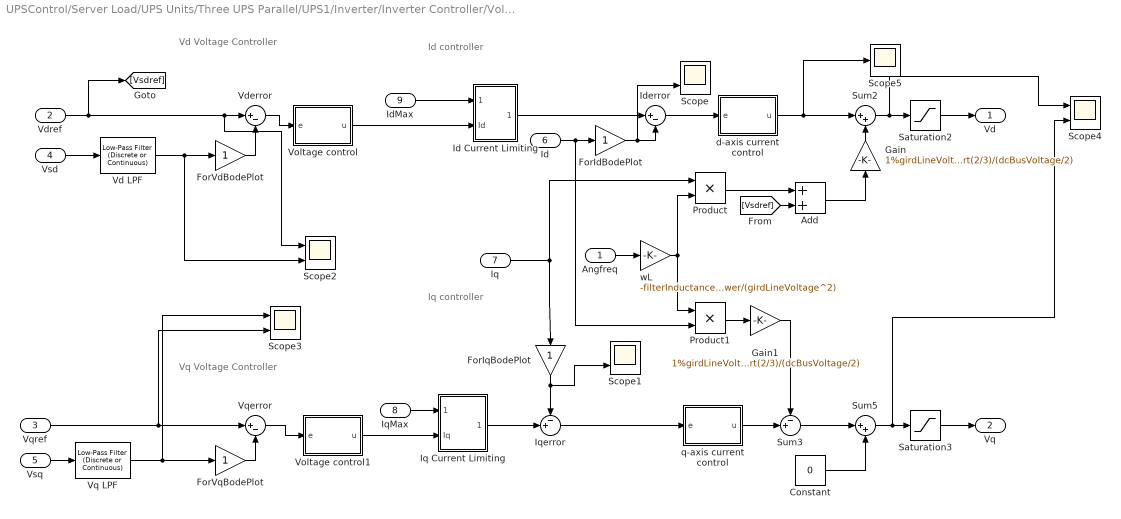
== system UPSControl/Server Load/UPS Units/Three UPS Parallel/UPS1/Inverter/Inverter Controller/VoltageCurrentControl/Controller ==
  note: Vq Voltage Controller
  note: Iq controller
  note: Vd Voltage Controller
  note: Id controller
  Angfreq : Inport
  Vdref : Inport  Port=2
  Vqref : Inport  Port=3
  Vsd : Inport  Port=4
  Vsq : Inport  Port=5
  Id : Inport  Port=6
  Iq : Inport  Port=7
  IqMax : Inport  Port=8
  IdMax : Inport  Port=9
  Add : Sum
  Constant : Constant  Value=0  SampleTime=currentControlTs
  ForIdBodePlot : Gain
  ForIqBodePlot : Gain
  ForVdBodePlot : Gain
  ForVqBodePlot : Gain
  Gain : Gain  Gain=1%girdLineVoltage*sqrt(2/3)/(dcBusVoltage/2)
  Gain1 : Gain  Gain=1%girdLineVoltage*sqrt(2/3)/(dcBusVoltage/2)
  Id Current Limiting : Subsystem
  Iderror : Sum  Inputs=|+-
  Iq Current Limiting : Subsystem
  Iqerror : Sum  Inputs=-+|
  Product : Product
  Product1 : Product
  Saturation2 : Saturate  UpperLimit=1.5  LowerLimit=-1.5
  Saturation3 : Saturate  UpperLimit=1.5  LowerLimit=-1.5
  Scope{,1..4} (5 alike) : Scope  NumInputPorts=2
      Scope settings: ActiveDisplayYMinimum=-1.8047219913264509  ActiveDisplayYMaximum=2.2005246657029387
      Scope1 settings: ActiveDisplayYMinimum=-0.5206159009733754  ActiveDisplayYMaximum=0.33911481242712255
      Scope2 settings: ActiveDisplayYMinimum=0.96150509431475939  ActiveDisplayYMaximum=1.0462950020078787
      Scope3 settings: ActiveDisplayYMinimum=-0.076556048576057134  ActiveDisplayYMaximum=0.019624633196700866
      Scope4 settings: ActiveDisplayYMinimum=-0.18956095761758107  ActiveDisplayYMaximum=1.4204991580589943  DataLoggingVariableName=ScopeData41
  Scope5 : Scope
      settings: ActiveDisplayYMinimum=-1  ActiveDisplayYMaximum=1  DataLoggingVariableName=ScopeData42
  Sum2 : Sum  Inputs=|++
  Sum3 : Sum  Inputs=-+|
  Sum5 : Sum  Inputs=|++
  Vd LPF : eeGeneralControl/Low-Pass Filter (Discrete or Continuous)  K=1  T=vdvqLPFTimeConst  B=inf  A=-inf  init_option=Specify as parameter  x0=0  Ts=voltControlTs
  Vderror : Sum  Inputs=|+-
  Voltage control : Subsystem
  Voltage control1 : Subsystem
  Vq LPF : eeGeneralControl/Low-Pass Filter (Discrete or Continuous)  K=1  T=vdvqLPFTimeConst  B=inf  A=-inf  init_option=Inherited from block input  x0=0  Ts=voltControlTs
  Vqerror : Sum  Inputs=|+-
  d-axis current control : Subsystem
  q-axis current control : Subsystem
  wL : Gain  Gain=-filterInductance*power/(girdLineVoltage^2)
  Vd : Outport  VectorParamsAs1DForOutWhenUnconnected=off
  Vq : Outport  Port=2  VectorParamsAs1DForOutWhenUnconnected=off
  wires:
  Vdref/1 -> [Vsdref], Vderror/1, Scope2/1
  Vq LPF/1 -> ForVqBodePlot/1, Scope3/1
  Vd LPF/1 -> ForVdBodePlot/1, Scope2/2
  ForIqBodePlot/1 -> Iqerror/1, Scope1/2
  ForIdBodePlot/1 -> Iderror/2, Scope/2
  ForVqBodePlot/1 -> Vqerror/2
  ForVdBodePlot/1 -> Vderror/2
  Vsd/1 -> Vd LPF/1
  Gain/1 -> Sum2/2
  Add/1 -> Gain/1
  [Vsdref] -> Add/2
  Gain1/1 -> Sum3/1
  Vqerror/1 -> Voltage control1/1(e)
  Vqref/1 -> Vqerror/1, Scope3/2
  Vderror/1 -> Voltage control/1(e)
  Id/1 -> ForIdBodePlot/1, Product1/2
  Vsq/1 -> Vq LPF/1
  Sum5/1 -> Scope4/2, Saturation3/1
  Sum3/1 -> Sum5/1
  q-axis current control/1(u) -> Sum3/2
  Sum2/1 -> Scope4/1, Saturation2/1
  d-axis current control/1(u) -> Scope5/1, Sum2/1
  Product/1 -> Add/1
  Product1/1 -> Gain1/1
  Saturation2/1 -> Vd/1
  Saturation3/1 -> Vq/1
  Iderror/1 -> d-axis current control/1(e)
  Constant/1 -> Sum5/2
  Angfreq/1 -> wL/1
  wL/1 -> Product/2, Product1/1
  Iqerror/1 -> q-axis current control/1(e)
  Iq/1 -> Product/1, ForIqBodePlot/1
  IdMax/1 -> Id Current Limiting/1(Imax)
  IqMax/1 -> Iq Current Limiting/1(Imax)
  Voltage control/1(u) -> Id Current Limiting/2(Id)
  Id Current Limiting/1(Idref) -> Iderror/1
  Voltage control1/1(u) -> Iq Current Limiting/2(Iq)
  Iq Current Limiting/1(Iqref) -> Iqerror/2

== system UPSControl/Server Load/UPS Units/Three UPS Parallel/UPS1/Inverter/Inverter Controller/VoltageCurrentControl/Modulation Signal ==
  Vd : Inport
  Vq : Inport  Port=2
  Angle : Inport  Port=3
  Constant : Constant  Value=0
  Constant1 : Constant  Value=1.05
  Inverse Park Transform : eeTransforms/Inverse Park Transform  AxisAlignment=D-axis  PowerInvariant=off
  Mux1 : Mux  Inputs=3
  Saturation : Saturate  UpperLimit=1.2  LowerLimit=-1.2
  Saturation1 : Saturate
  Saturation2 : Saturate  UpperLimit=1  LowerLimit=-1
  Scope : Scope  NumInputPorts=2
      settings: ActiveDisplayYMinimum=-1  ActiveDisplayYMaximum=1  DataLoggingVariableName=ScopeData9
  Scope1 : Scope
      settings: ActiveDisplayYMinimum=-1  ActiveDisplayYMaximum=1
  Scope2 : Scope
      settings: ActiveDisplayYMinimum=-1.25  ActiveDisplayYMaximum=1.25  DataLoggingVariableName=ScopeData47
  mabc : Outport  VectorParamsAs1DForOutWhenUnconnected=off
  wires:
  Vq/1 -> Saturation1/1, Scope/2
  Vd/1 -> Saturation/1, Scope/1
  Constant/1 -> Mux1/3
  Saturation2/1 -> Scope2/1, mabc/1
  Angle/1 -> Inverse Park Transform/2, Scope1/1
  Mux1/1 -> Inverse Park Transform/1
  Inverse Park Transform/1 -> Saturation2/1
  Saturation/1 -> Mux1/1
  Saturation1/1 -> Mux1/2

== system UPSControl/Server Load/UPS Units/Three UPS Parallel/UPS1/Rectifier/PFC Rectifier Controller/Current Controller/Id and Iq Controller ==
  idRef : Inport
  iqRef : Inport  Port=2
  IdSens : Inport  Port=3
  iqSens : Inport  Port=4
  vd : Inport  Port=5
  vq : Inport  Port=6
  Reset : Inport  Port=7
  Constant4 : Constant  Value=0  SampleTime=Ts
  Gain1 : Gain  Gain=2*1*pi*Freq*L/BaseImpedance
  Gain2 : Gain  Gain=2*1*pi*Freq*L/BaseImpedance
  IdPID : slpidlib/PID Controller  Controller=PID  Form=Parallel  TimeDomain=Discrete-time  UseExternalTs=off  SampleTime=Ts  IntegratorMethod=Forward Euler  FilterMethod=Forward Euler  ControllerParametersSource=internal  P=KpdCurrent  I=KidCurrent  UseKiTs=off  D=KddCurrent  UseExternalDerivativeSource=off  N=NdCurrent  UseFilter=on  TunerSelectOption=Transfer Function Based (PID Tuner App)  InitialConditionSource=internal  InitialConditionForIntegrator=0  InitialConditionForFilter=0  DifferentiatorICPrevScaledInput=0  ExternalReset=falling  TrackingMode=off  Kt=1  LimitOutput=on  SatLimitsSource=internal  UpperSaturationLimit=IdControlUpperLimit  LowerSaturationLimit=IdControlLowerLimit  LinearizeAsGain=on  AntiWindupMode=clamping  Kb=1  LimitIntegrator=on  UpperIntegratorSaturationLimit=IdControlUpperLimit  LowerIntegratorSaturationLimit=IdControlLowerLimit  POutMin=[]  POutMax=[]  IOutMin=[]  IOutMax=[]  DOutMin=[]  DOutMax=[]  NOutMin=[]  NOutMax=[]  SumOutMin=[]  SumOutMax=[]  SaturationOutMin=[]  SaturationOutMax=[]  PParamMin=[]  PParamMax=[]  IParamMin=[]  IParamMax=[]  DParamMin=[]  DParamMax=[]  NParamMin=[]  NParamMax=[]  KbParamMin=[]  KbParamMax=[]  KtParamMin=[]  KtParamMax=[]  KbOutMin=[]  KbOutMax=[]  KtOutMin=[]  KtOutMax=[]  IntegratorOutMin=[]  IntegratorOutMax=[]  FilterOutMin=[]  FilterOutMax=[]  SumI1OutMin=[]  SumI1OutMax=[]  SumI2OutMin=[]  SumI2OutMax=[]  SumI3OutMin=[]  SumI3OutMax=[]  SumI4OutMin=[]  SumI4OutMax=[]  SumDOutMin=[]  SumDOutMax=[]  DifferentiatorOutMin=[]  DifferentiatorOutMax=[]  FilterDiffOutCoefMin=[]  FilterDiffOutCoefMax=[]  ReciprocalOutMin=[]  ReciprocalOutMax=[]  SumDenOutMin=[]  SumDenOutMax=[]  SumNumOutMin=[]  SumNumOutMax=[]  DivideOutMin=[]  DivideOutMax=[]  UdiffTsProdOutMin=[]  UdiffTsProdOutMax=[]  NTsProdOutMin=[]  NTsProdOutMax=[]  UintegralTsProdOutMin=[]  UintegralTsProdOutMax=[]  UngainTsProdOutMin=[]  UngainTsProdOutMax=[]  ClampingZeroOutDataTypeStr=Inherit: Inherit via back propagation  ClampingZeroOutMin=[]  ClampingZeroOutMax=[]  FilterDenConstantOutDataTypeStr=Inherit: Inherit via back propagation  FilterDenConstantOutMin=[]  FilterDenConstantOutMax=[]  PCopyOutDataTypeStr=Inherit: Inherit via back propagation  PCopyOutMin=[]  PCopyOutMax=[]  NCopyOutDataTypeStr=Inherit: Inherit via back propagation  NCopyOutMin=[]  NCopyOutMax=[]  IntegratorContinuousStateAttributes=''  IntegratorStateMustResolveToSignalObject=off  IntegratorRTWStateStorageClass=Auto  FilterContinuousStateAttributes=''  FilterStateMustResolveToSignalObject=off  FilterRTWStateStorageClass=Auto  ParallelPVariant=InternalParameters  IdealPVariant=Disabled  IVariant=InternalParameters  DVariant=InternalParameters  IntegratorVariant=Discrete  SatVariant=Enabled  AWVariant=DiscClampingParallel  PCopyVariant=Disabled  TRVariant=Disabled  FdbkBlocksVariant=Forward  IdealPFdbkVariant=Disabled  SatFdbkVariant=Disabled  DerivativeFilterVariant=ForwardEulerFilter  NVariant=InternalParameters  NCopyVariant=Disabled  FilterICVariant=InternalICsFilter  IntegratorICVariant=InternalICs  ExternalResetVariant=ExternalReset  TRSumVariant=Passthrough  SumFdbkVariant=Disabled  SumVariant=Sum_PID  TsampFilterVariant=InternalTs  TsampNgainVariant=Passthrough  TsampIntegralVariant=Disabled_SignalSpec  ExternalSaturationOutDataTypeStr=Inherit: Same as second input  DerivativeSourceVariant=ErrorSignal  PreIntVariant=InternalPreInt
  IqPID : slpidlib/PID Controller  Controller=PID  Form=Parallel  TimeDomain=Discrete-time  UseExternalTs=off  SampleTime=Ts  IntegratorMethod=Forward Euler  FilterMethod=Forward Euler  ControllerParametersSource=internal  P=KpqCurrent  I=KiqCurrent  UseKiTs=off  D=KdqCurrent  UseExternalDerivativeSource=off  N=NdCurrent  UseFilter=on  TunerSelectOption=Transfer Function Based (PID Tuner App)  InitialConditionSource=internal  InitialConditionForIntegrator=0  InitialConditionForFilter=0  DifferentiatorICPrevScaledInput=0  ExternalReset=falling  TrackingMode=off  Kt=1  LimitOutput=on  SatLimitsSource=internal  UpperSaturationLimit=IqControlUpperLimit  LowerSaturationLimit=IqControlLowerLimit  LinearizeAsGain=on  AntiWindupMode=clamping  Kb=1  LimitIntegrator=on  UpperIntegratorSaturationLimit=IqControlUpperLimit  LowerIntegratorSaturationLimit=IqControlLowerLimit  POutMin=[]  POutMax=[]  IOutMin=[]  IOutMax=[]  DOutMin=[]  DOutMax=[]  NOutMin=[]  NOutMax=[]  SumOutMin=[]  SumOutMax=[]  SaturationOutMin=[]  SaturationOutMax=[]  PParamMin=[]  PParamMax=[]  IParamMin=[]  IParamMax=[]  DParamMin=[]  DParamMax=[]  NParamMin=[]  NParamMax=[]  KbParamMin=[]  KbParamMax=[]  KtParamMin=[]  KtParamMax=[]  KbOutMin=[]  KbOutMax=[]  KtOutMin=[]  KtOutMax=[]  IntegratorOutMin=[]  IntegratorOutMax=[]  FilterOutMin=[]  FilterOutMax=[]  SumI1OutMin=[]  SumI1OutMax=[]  SumI2OutMin=[]  SumI2OutMax=[]  SumI3OutMin=[]  SumI3OutMax=[]  SumI4OutMin=[]  SumI4OutMax=[]  SumDOutMin=[]  SumDOutMax=[]  DifferentiatorOutMin=[]  DifferentiatorOutMax=[]  FilterDiffOutCoefMin=[]  FilterDiffOutCoefMax=[]  ReciprocalOutMin=[]  ReciprocalOutMax=[]  SumDenOutMin=[]  SumDenOutMax=[]  SumNumOutMin=[]  SumNumOutMax=[]  DivideOutMin=[]  DivideOutMax=[]  UdiffTsProdOutMin=[]  UdiffTsProdOutMax=[]  NTsProdOutMin=[]  NTsProdOutMax=[]  UintegralTsProdOutMin=[]  UintegralTsProdOutMax=[]  UngainTsProdOutMin=[]  UngainTsProdOutMax=[]  ClampingZeroOutDataTypeStr=Inherit: Inherit via back propagation  ClampingZeroOutMin=[]  ClampingZeroOutMax=[]  FilterDenConstantOutDataTypeStr=Inherit: Inherit via back propagation  FilterDenConstantOutMin=[]  FilterDenConstantOutMax=[]  PCopyOutDataTypeStr=Inherit: Inherit via back propagation  PCopyOutMin=[]  PCopyOutMax=[]  NCopyOutDataTypeStr=Inherit: Inherit via back propagation  NCopyOutMin=[]  NCopyOutMax=[]  IntegratorContinuousStateAttributes=''  IntegratorStateMustResolveToSignalObject=off  IntegratorRTWStateStorageClass=Auto  FilterContinuousStateAttributes=''  FilterStateMustResolveToSignalObject=off  FilterRTWStateStorageClass=Auto  ParallelPVariant=InternalParameters  IdealPVariant=Disabled  IVariant=InternalParameters  DVariant=InternalParameters  IntegratorVariant=Discrete  SatVariant=Enabled  AWVariant=DiscClampingParallel  PCopyVariant=Disabled  TRVariant=Disabled  FdbkBlocksVariant=Forward  IdealPFdbkVariant=Disabled  SatFdbkVariant=Disabled  DerivativeFilterVariant=ForwardEulerFilter  NVariant=InternalParameters  NCopyVariant=Disabled  FilterICVariant=InternalICsFilter  IntegratorICVariant=InternalICs  ExternalResetVariant=ExternalReset  TRSumVariant=Passthrough  SumFdbkVariant=Disabled  SumVariant=Sum_PID  TsampFilterVariant=InternalTs  TsampNgainVariant=Passthrough  TsampIntegralVariant=Disabled_SignalSpec  ExternalSaturationOutDataTypeStr=Inherit: Same as second input  DerivativeSourceVariant=ErrorSignal  PreIntVariant=InternalPreInt
  Mux1 : Mux  Inputs=3
  Sum1 : Sum  Inputs=|+-
  Sum2 : Sum  Inputs=|+-+
  Sum4 : Sum  Inputs=|--+
  Sum5 : Sum  Inputs=|+-
  vdqoRef : Outport
  IdCntrlError : Outport  Port=2
  IqCntrlError : Outport  Port=3
  wires:
  iqRef/1 -> Sum5/1
  Mux1/1 -> vdqoRef/1
  idRef/1 -> Sum1/1
  IqPID/1 -> Sum4/2
  IdSens/1 -> Gain1/1, Sum1/2
  Sum1/1 -> IdPID/1, IdCntrlError/1
  vd/1 -> Sum2/1
  IdPID/1 -> Sum2/2
  Gain2/1 -> Sum2/3
  Gain1/1 -> Sum4/1
  vq/1 -> Sum4/3
  iqSens/1 -> Gain2/1, Sum5/2
  Sum2/1 -> Mux1/1
  Sum4/1 -> Mux1/2
  Sum5/1 -> IqPID/1, IqCntrlError/1
  Constant4/1 -> Mux1/3
  Reset/1 -> IqPID/2, IdPID/2

== system UPSControl/Server Load/UPS Units/Three UPS Parallel/UPS1/Rectifier/PFC Rectifier Controller/DC Voltage Controller and Current Reference/Iq Reference ==
  V_mag : Inport
  Q_ref : Inport  Port=2
  Divide2 : Product  Inputs=*/
  iq_ref : Outport
  wires:
  V_mag/1 -> Divide2/2
  Q_ref/1 -> Divide2/1
  Divide2/1 -> iq_ref/1

== system UPSControl/Server Load/UPS Units/Three UPS Parallel/UPS1/Rectifier/PFC Rectifier Controller/DC Voltage Controller and Current Reference/Voltage Controller ==
  Vdcref : Inport
  Vdcmeas : Inport  Port=2
  Reset : Inport  Port=3
  Gain : Gain  Gain=1/BaseVdc
  Saturation : Saturate  UpperLimit=IdRefUpperLimit  LowerLimit=0
  Sum : Sum  Inputs=|+-
  Voltage control : Subsystem
  Id : Outport
  wires:
  Sum/1 -> Gain/1
  Gain/1 -> Voltage control/1(e)
  Vdcmeas/1 -> Sum/2
  Vdcref/1 -> Sum/1
  Voltage control/1(u) -> Saturation/1
  Saturation/1 -> Id/1
  Reset/1 -> Voltage control/2(Reset)
